simulink model "controller"  (R2018b)
settings: Solver=VariableStepAuto  StartTime=0.0  StopTime=Endtime  RelTol=1e-3
values from neighbouring files (symbols this model uses):
  alpha_A = (2^n - 1)/(V_A_max - V_A_min)    (= 204.6)    [ADC_sim.m]    (also in controller_sim.m)
  alpha_i = 5/37.5    (= 0.133333333333)    [controller_sim.m]
  alpha_T = 1.5/1000    (= 0.0015)    [controller_sim.m]
  d_i_d = (2^n-1)/60    (= 17.05)    [controller_sim.m]
  d_N_d = (2^n-1)/60    (= 17.05)    [controller_sim.m]
  m = 8    [controller_sim.m]    (also in pulse_gen_sim.m)
  smp = 0.001    [ADC_sim.m]    (also in controller_sim.m; pulse_gen_sim.m = 0.01)
  u_max = 100    [controller_sim.m]
  u_min = 0    [controller_sim.m]
  V_A_min = 0    [ADC_sim.m]    (also in controller_sim.m)
libraries: simulink x2
settings Model: Creator=nharada  LastModifiedBy=nharada

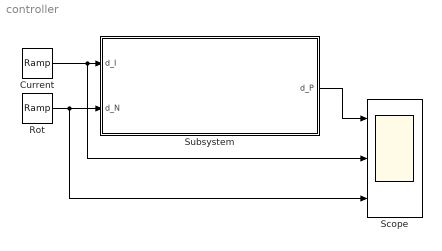
== system controller ==
  Current : simulink/Sources/Ramp  slope=d_i_d  start=0  InitialOutput=0
  "Rot " : simulink/Sources/Ramp  slope=d_N_d  start=0  InitialOutput=0
  Scope : Scope  NumInputPorts=3
  Subsystem : Subsystem
  wires:
  Current/1 -> Scope/2, Subsystem/1(d_I)
  "Rot "/1 -> Subsystem/2(d_N), Scope/3
  Subsystem/1(d_P) -> Scope/1

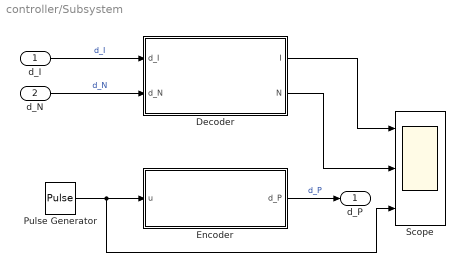
== system controller/Subsystem ==
  d_I : Inport
  d_N : Inport  Port=2
  Decoder : Subsystem
  Encoder : Subsystem
  Pulse Generator : DiscretePulseGenerator  PulseType=Time based  Amplitude=100  Period=30  PulseWidth=50
  Scope : Scope  NumInputPorts=3
  d_P : Outport
  wires:
  Pulse Generator/1 -> Scope/3, Encoder/1(u)
  Decoder/2(N) -> Scope/2
  d_N/1 -> Decoder/2(d_N)  "d_N"
  Decoder/1(I) -> Scope/1
  d_I/1 -> Decoder/1(d_I)  "d_I"
  Encoder/1(d_P) -> d_P/1  "d_P"

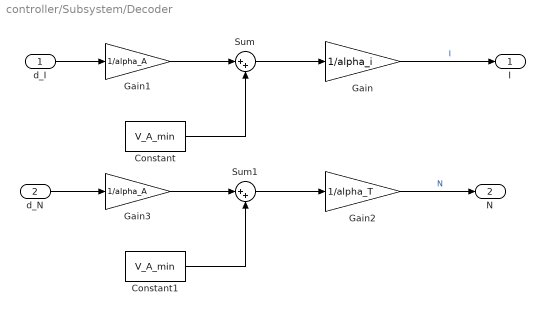
== system controller/Subsystem/Decoder ==
  d_I : Inport
  d_N : Inport  Port=2
  Constant : Constant  Value=V_A_min  SampleTime=smp
  Constant1 : Constant  Value=V_A_min  SampleTime=smp
  Gain : Gain  Gain=1/alpha_i
  Gain1 : Gain  Gain=1/alpha_A
  Gain2 : Gain  Gain=1/alpha_T
  Gain3 : Gain  Gain=1/alpha_A
  Sum : Sum  Inputs=|++
  Sum1 : Sum  Inputs=|++
  I : Outport
  N : Outport  Port=2
  wires:
  Gain2/1 -> N/1  "N"
  Constant1/1 -> Sum1/2
  Gain/1 -> I/1  "I"
  Gain1/1 -> Sum/1
  d_N/1 -> Gain3/1
  Gain3/1 -> Sum1/1
  d_I/1 -> Gain1/1
  Constant/1 -> Sum/2
  Sum/1 -> Gain/1
  Sum1/1 -> Gain2/1

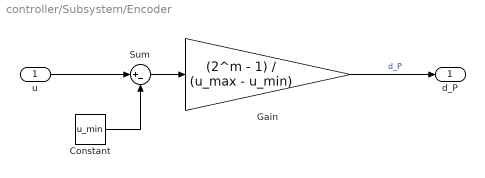
== system controller/Subsystem/Encoder ==
  u : Inport
  Constant : Constant  Value=u_min  SampleTime=smp
  Gain : Gain  Gain=(2^m - 1) / (u_max - u_min)
  Sum : Sum  Inputs=|+-
  d_P : Outport
  wires:
  Sum/1 -> Gain/1
  Constant/1 -> Sum/2
  u/1 -> Sum/1
  Gain/1 -> d_P/1  "d_P"
